simulink model "s_heli3d"  (R2022b)
settings: Solver=FixedStepAuto  StartTime=0.0  StopTime=50  FixedStep=0.05  RelTol=1e-3  EnableMultiTasking=on
values from neighbouring files (symbols this model uses):
  CMD_RATE_LIMIT = 45.0 * pi / 180    (= 0.785398163397)    [setup_lab_heli_3d.m]
  K = zeros(2,6)    [setup_lab_heli_3d.m]
  K_AMP = 3    [setup_lab_heli_3d.m]
  SAT_INT_ERR_ELEV = 7.5    [setup_lab_heli_3d.m]
  SAT_INT_ERR_TRAVEL = 7.5    [setup_lab_heli_3d.m]
  VMAX_AMP = 24    [setup_lab_heli_3d.m]
  VMAX_DAC = 10    [setup_lab_heli_3d.m]
undefined symbols (not defined in the file or in its folder): A, B, F, G, H, L_input, L_states, N, u_max_hat, u_min_hat, x_max_hat, x_min_hat
libraries: simulink_extras x6
settings Model: ExtModeTrigDuration=5000  Creator=MLevis  LastModifiedBy=START
settings SolverCC: AlgebraicLoopSolver=TrustRegion  PositivePriorityOrder=on
settings DataIOCC: LimitDataPoints=on  SaveFormat=Array  SignalLoggingSaveFormat=ModelDataLogs  ReturnWorkspaceOutputs=off
settings OptimizationCC: BooleanDataType=off  OptimizeBlockIOStorage=off  BufferReuse=off  ExpressionFolding=off  ExpressionDepthLimit=2147483647  LocalBlockOutputs=off  InitFltsAndDblsToZero=on
settings DebuggingCC: SaveWithParameterizedLinksMsg=none  UnderspecifiedInitializationDetection=Classic  MergeDetectMultiDrivingBlocksExec=none  SignalResolutionControl=TryResolveAllWithWarning  SolverPrmCheckMsg=warning  MultiTaskDSMMsg=warning  MultiTaskCondExecSysMsg=none  FcnCallInpInsideContextMsg=warning  UnconnectedInputMsg=warning  UnconnectedOutputMsg=warning  UnconnectedLineMsg=warning  StateNameClashWarn=warning  SFUnexpectedBacktrackingDiag=warning  SFNoUnconditionalDefaultTransitionDiag=warning  SFExecutionAtInitializationDiag=none  SFMachineParentedDataDiag=warning  ArithmeticOperatorsInVariantConditions=warning
settings HardwareCC: ProdBitPerPointer=32  ProdBitPerSizeT=32  ProdBitPerPtrDiffT=32  ProdWordSize=32  ProdHWDeviceType=Intel->x86-32 (Windows32)
settings ModelReferenceCC: EnableRefExpFcnMdlSchedulingChecks=on  PropagateSignalLabelsOutOfModel=off
settings RTWCC: Description=QUARC Win32 Target Using Toolchain  SystemTargetFile=quarc_windows.tlc  TemplateMakefile=quarc_default_tmf  Toolchain=QUARC windows | nmake (64-bit Windows)  BuildConfiguration=Faster Runs  DLArmComputeVersion=19.05
settings CodeAppCC: StateflowObjectComments=on
settings STFCustomTargetCC: ConcurrentExecutionCompliant=on  GRTInterface=on  UseToolchainInfoCompliant=on  SystemTargetFile=quarc_windows.tlc
settings GRTTargetCC: TargetLangStandard=C89/C90 (ANSI)  ParMdlRefBuildCompliant=off  CompOptLevelCompliant=off  CombineOutputUpdateFcns=off  MatFileLogging=off  CPPClassGenCompliant=off  GRTInterface=on  ExtMode=on  ExtModeMexFile=quarc_comm
settings ConfigComp: CovMetricSettings=dw  CovSaveCumulativeToWorkspaceVar=on  CovSaveSingleToWorkspaceVar=on

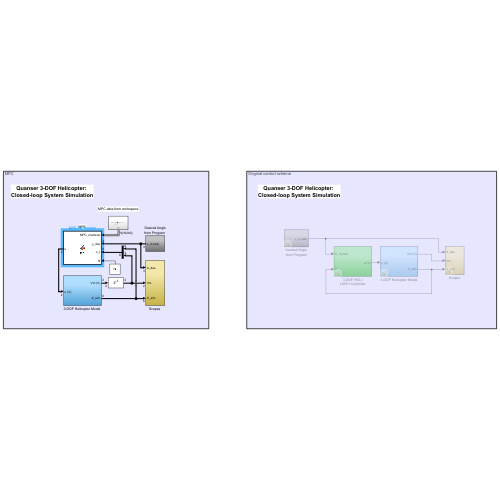
[thumbnail: Simulink's stored preview of the top-level diagram]
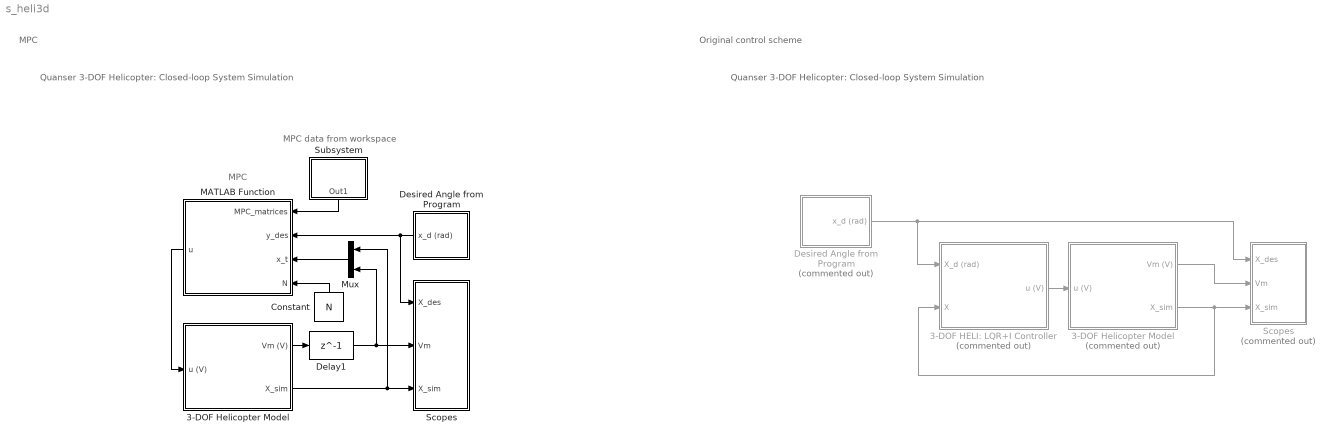
== system s_heli3d ==
  note: Original control scheme
  note: MPC
  note: MPC data from workspace
  note: MPC
  note: Quanser 3-DOF Helicopter:
      | Closed-loop System Simulation
  note: Quanser 3-DOF Helicopter:
      | Closed-loop System Simulation
  3-DOF HELI: LQR+I Controller : Subsystem  Commented=on  AncestorBlock=heli_2d_lib/2DOF HELI: FF+LQR+I Controller
      settings: LibrarySourceBlock=|
      | heli_2d_lib/2DOF HELI:
      | FF+LQR+I Controller
  3-DOF Helicopter Model : Subsystem  Commented=on
  "3-DOF Helicopter Model " : Subsystem
  Constant : Constant  Value=N
  Delay1 : Delay  DelayLength=1  InitialCondition=0
  Desired Angle from Program : Subsystem  Commented=on
  "Desired Angle from Program " : Subsystem
  MATLAB Function : MATLAB Function  Tag=MPC  Description=MPC  TreatAsAtomicUnit=on
  Mux : Mux  Inputs=2
  Scopes : Subsystem  Commented=on
  "Scopes " : Subsystem
  Subsystem : Subsystem
  wires:
  Desired Angle from Program/1(x_d (rad)) -> Scopes/1(X_des), 3-DOF HELI: LQR+I Controller/1(X_d (rad))
  3-DOF HELI: LQR+I Controller/1(u (V)) -> 3-DOF Helicopter Model/1(u (V))
  3-DOF Helicopter Model/2(X_sim) -> Scopes/3(X_sim), 3-DOF HELI: LQR+I Controller/2(X)
  3-DOF Helicopter Model/1(Vm (V)) -> Scopes/2(Vm)
  Mux/1 -> MATLAB Function/3(x_t)
  MATLAB Function/1(u) -> "3-DOF Helicopter Model "/1(u (V))
  "3-DOF Helicopter Model "/2(X_sim) -> Mux/1, "Scopes "/3(X_sim)
  "3-DOF Helicopter Model "/1(Vm (V)) -> Delay1/1
  "Desired Angle from Program "/1(x_d (rad)) -> MATLAB Function/2(y_des), "Scopes "/1(X_des)
  Subsystem/1(Out1) -> MATLAB Function/1(MPC_matrices)
  Constant/1 -> MATLAB Function/4(N)
  Delay1/1 -> Mux/2, "Scopes "/2(Vm)

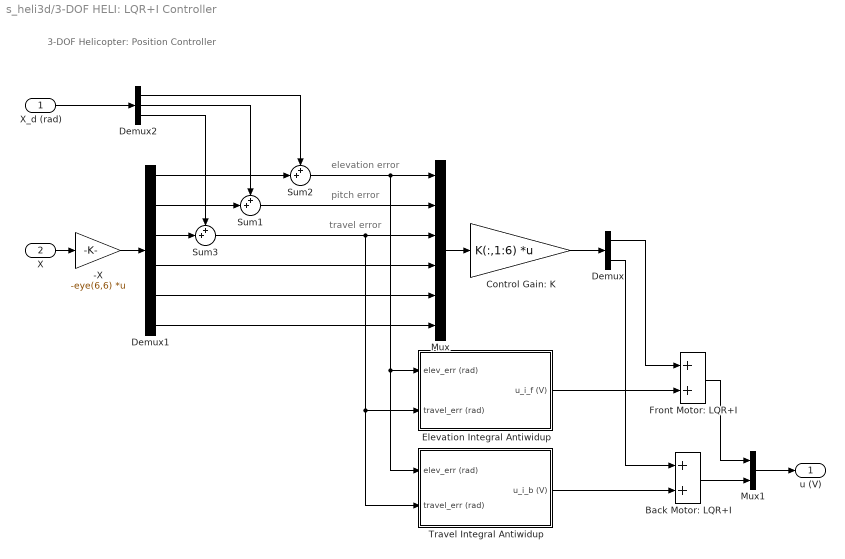
== system s_heli3d/3-DOF HELI: LQR+I Controller ==
  note: elevation error
  note: pitch error
  note: 3-DOF Helicopter: Position Controller
  note: travel error
  X_d (rad) : Inport
  X : Inport  Port=2
  -X : Gain  Gain=-eye(6,6)  Multiplication=Matrix(K*u)
  Back Motor: LQR+I : Sum
  Control Gain: K : Gain  Gain=K(:,1:6)  Multiplication=Matrix(K*u)
  Demux : Demux  Outputs=2
  Demux1 : Demux  Outputs=6
  Demux2 : Demux  Outputs=3
  Elevation Integral Antiwidup : Subsystem
  Front Motor: LQR+I : Sum
  Mux : Mux  Inputs=6
  Mux1 : Mux  Inputs=2
  Sum1 : Sum  Inputs=++|
  Sum2 : Sum  Inputs=++|
  Sum3 : Sum  Inputs=++|
  Travel Integral Antiwidup : Subsystem
  u (V) : Outport
  wires:
  Back Motor: LQR+I/1 -> Mux1/2
  Demux/1 -> Front Motor: LQR+I/1
  Demux/2 -> Back Motor: LQR+I/1
  Travel Integral Antiwidup/1(u_i_b (V)) -> Back Motor: LQR+I/2
  Elevation Integral Antiwidup/1(u_i_f (V)) -> Front Motor: LQR+I/2
  Demux1/2 -> Sum1/2
  Demux2/2 -> Sum1/1
  Demux2/1 -> Sum2/1
  X_d (rad)/1 -> Demux2/1
  Sum2/1 -> Mux/1, Elevation Integral Antiwidup/1(elev_err (rad)), Travel Integral Antiwidup/1(elev_err (rad))
  Demux1/1 -> Sum2/2
  X/1 -> -X/1
  Sum1/1 -> Mux/2
  -X/1 -> Demux1/1
  Mux/1 -> Control Gain: K/1
  Demux1/4 -> Mux/4
  Demux2/3 -> Sum3/1
  Demux1/3 -> Sum3/2
  Sum3/1 -> Mux/3, Elevation Integral Antiwidup/2(travel_err (rad)), Travel Integral Antiwidup/2(travel_err (rad))
  Demux1/5 -> Mux/5
  Demux1/6 -> Mux/6
  Control Gain: K/1 -> Demux/1
  Mux1/1 -> u (V)/1
  Front Motor: LQR+I/1 -> Mux1/1

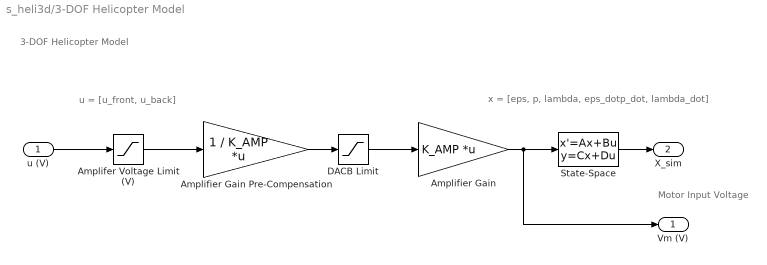
== system s_heli3d/3-DOF Helicopter Model ==
  note: x = [eps, p, lambda, eps_dotp_dot, lambda_dot]
  note: u = [u_front, u_back]
  note: Motor Input Voltage
  note: 3-DOF Helicopter Model
  u (V) : Inport
  Amplifer Voltage Limit (V) : Saturate  UpperLimit=VMAX_AMP  LowerLimit=-VMAX_AMP
  Amplifier Gain : Gain  Gain=K_AMP  Multiplication=Matrix(K*u)  SaturateOnIntegerOverflow=on  OutDataTypeStr=Inherit: Same as input  ParamDataTypeStr=Inherit: Same as input
  Amplifier Gain Pre-Compensation : Gain  Gain=1 / K_AMP  Multiplication=Matrix(K*u)  SaturateOnIntegerOverflow=on  OutDataTypeStr=Inherit: Same as input  ParamDataTypeStr=Inherit: Same as input
  DACB Limit : Saturate  UpperLimit=VMAX_DAC  LowerLimit=-VMAX_DAC
  State-Space : StateSpace  A=A  B=B  C=eye(6,6)  D=zeros(6,2)  InitialCondition=0
  Vm (V) : Outport
  X_sim : Outport  Port=2
  wires:
  u (V)/1 -> Amplifer Voltage Limit (V)/1
  Amplifier Gain/1 -> Vm (V)/1, State-Space/1
  State-Space/1 -> X_sim/1
  Amplifer Voltage Limit (V)/1 -> Amplifier Gain Pre-Compensation/1
  Amplifier Gain Pre-Compensation/1 -> DACB Limit/1
  DACB Limit/1 -> Amplifier Gain/1

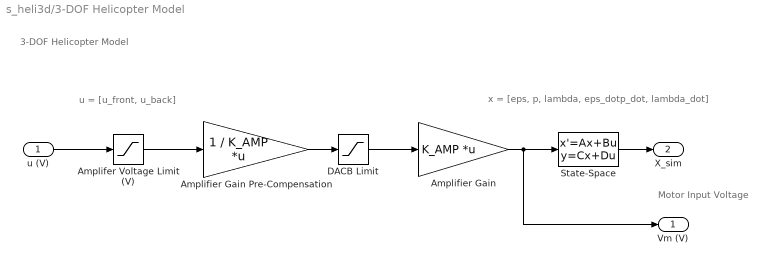
== system s_heli3d/3-DOF Helicopter Model  ==
  note: x = [eps, p, lambda, eps_dotp_dot, lambda_dot]
  note: u = [u_front, u_back]
  note: Motor Input Voltage
  note: 3-DOF Helicopter Model
  u (V) : Inport
  Amplifer Voltage Limit (V) : Saturate  UpperLimit=VMAX_AMP  LowerLimit=-VMAX_AMP
  Amplifier Gain : Gain  Gain=K_AMP  Multiplication=Matrix(K*u)  SaturateOnIntegerOverflow=on  OutDataTypeStr=Inherit: Same as input  ParamDataTypeStr=Inherit: Same as input
  Amplifier Gain Pre-Compensation : Gain  Gain=1 / K_AMP  Multiplication=Matrix(K*u)  SaturateOnIntegerOverflow=on  OutDataTypeStr=Inherit: Same as input  ParamDataTypeStr=Inherit: Same as input
  DACB Limit : Saturate  UpperLimit=VMAX_DAC  LowerLimit=-VMAX_DAC
  State-Space : StateSpace  A=A  B=B  C=eye(6,6)  D=zeros(6,2)  InitialCondition=0
  Vm (V) : Outport
  X_sim : Outport  Port=2
  wires:
  u (V)/1 -> Amplifer Voltage Limit (V)/1
  Amplifier Gain/1 -> Vm (V)/1, State-Space/1
  State-Space/1 -> X_sim/1
  Amplifer Voltage Limit (V)/1 -> Amplifier Gain Pre-Compensation/1
  Amplifier Gain Pre-Compensation/1 -> DACB Limit/1
  DACB Limit/1 -> Amplifier Gain/1

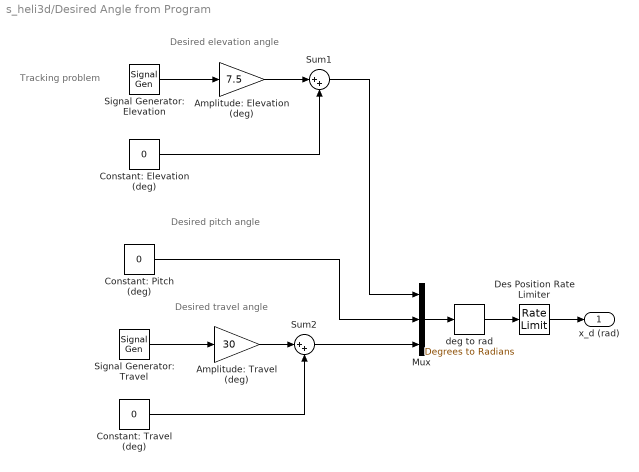
== system s_heli3d/Desired Angle from Program ==
  note: Tracking problem
  note: Desired elevation angle
  note: Desired travel angle
  note: Desired pitch angle
  Amplitude: Elevation (deg) : Gain  Gain=7.5
  Amplitude: Travel (deg) : Gain  Gain=30
  Constant: Elevation (deg) : Constant  Value=0
  Constant: Pitch (deg) : Constant  Value=0
  Constant: Travel (deg) : Constant  Value=0
  Des Position Rate Limiter : RateLimiter  RisingSlewLimit=CMD_RATE_LIMIT  FallingSlewLimit=-CMD_RATE_LIMIT  SampleTimeMode=inherited
  Mux : Mux  Inputs=3
  Signal Generator: Elevation : SignalGenerator  WaveForm=square  Frequency=0.04
  Signal Generator: Travel : SignalGenerator  WaveForm=square  Frequency=0.03
  Sum1 : Sum  Inputs=|++
  Sum2 : Sum  Inputs=|++
  deg to rad : simulink_extras/Transformations/Degrees to Radians
  x_d (rad) : Outport
  wires:
  Mux/1 -> deg to rad/1
  Constant: Elevation (deg)/1 -> Sum1/2
  Amplitude: Elevation (deg)/1 -> Sum1/1
  Signal Generator: Elevation/1 -> Amplitude: Elevation (deg)/1
  Constant: Travel (deg)/1 -> Sum2/2
  Amplitude: Travel (deg)/1 -> Sum2/1
  Signal Generator: Travel/1 -> Amplitude: Travel (deg)/1
  Sum2/1 -> Mux/3
  deg to rad/1 -> Des Position Rate Limiter/1
  Constant: Pitch (deg)/1 -> Mux/2
  Sum1/1 -> Mux/1
  Des Position Rate Limiter/1 -> x_d (rad)/1

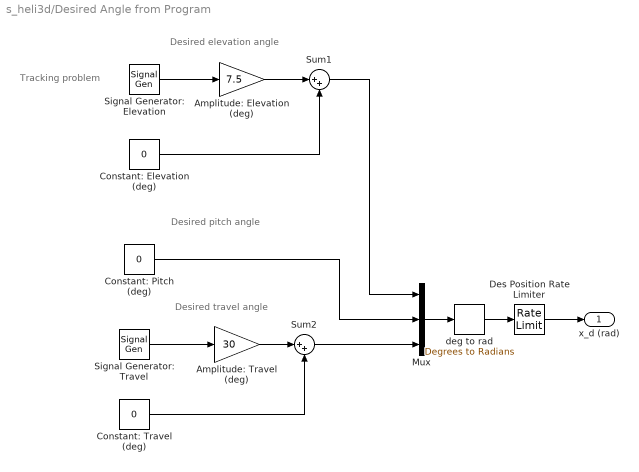
== system s_heli3d/Desired Angle from Program  ==
  note: Tracking problem
  note: Desired elevation angle
  note: Desired travel angle
  note: Desired pitch angle
  Amplitude: Elevation (deg) : Gain  Gain=7.5
  Amplitude: Travel (deg) : Gain  Gain=30
  Constant: Elevation (deg) : Constant  Value=0
  Constant: Pitch (deg) : Constant  Value=0
  Constant: Travel (deg) : Constant  Value=0
  Des Position Rate Limiter : RateLimiter  RisingSlewLimit=CMD_RATE_LIMIT  FallingSlewLimit=-CMD_RATE_LIMIT  SampleTimeMode=inherited
  Mux : Mux  Inputs=3
  Signal Generator: Elevation : SignalGenerator  WaveForm=square  Frequency=0.04
  Signal Generator: Travel : SignalGenerator  WaveForm=square  Frequency=0.03
  Sum1 : Sum  Inputs=|++
  Sum2 : Sum  Inputs=|++
  deg to rad : simulink_extras/Transformations/Degrees to Radians
  x_d (rad) : Outport
  wires:
  Mux/1 -> deg to rad/1
  Signal Generator: Elevation/1 -> Amplitude: Elevation (deg)/1
  Constant: Travel (deg)/1 -> Sum2/2
  Signal Generator: Travel/1 -> Amplitude: Travel (deg)/1
  Sum2/1 -> Mux/3
  Constant: Pitch (deg)/1 -> Mux/2
  Sum1/1 -> Mux/1
  Constant: Elevation (deg)/1 -> Sum1/2
  Amplitude: Elevation (deg)/1 -> Sum1/1
  deg to rad/1 -> Des Position Rate Limiter/1
  Des Position Rate Limiter/1 -> x_d (rad)/1
  Amplitude: Travel (deg)/1 -> Sum2/1

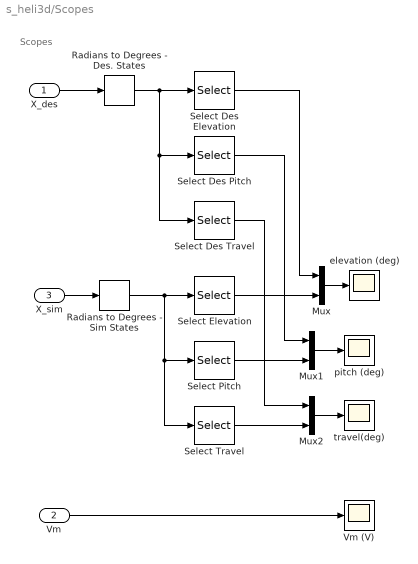
== system s_heli3d/Scopes ==
  note: Scopes
  X_des : Inport
  Vm : Inport  Port=2
  X_sim : Inport  Port=3
  Mux : Mux  Inputs=2
  Mux1 : Mux  Inputs=2
  Mux2 : Mux  Inputs=2
  Radians to Degrees - Des. States : simulink_extras/Transformations/Radians to Degrees
  Radians to Degrees - Sim States : simulink_extras/Transformations/Radians to Degrees
  Select Des Elevation : Selector  InputPortWidth=3  IndexOptions=Index vector (dialog)  Indices=1  OutputSizes=1
  Select Des Pitch : Selector  InputPortWidth=3  IndexOptions=Index vector (dialog)  Indices=2  OutputSizes=1
  Select Des Travel : Selector  InputPortWidth=3  IndexOptions=Index vector (dialog)  Indices=3  OutputSizes=1
  Select Elevation : Selector  InputPortWidth=6  IndexOptions=Index vector (dialog)  Indices=1  OutputSizes=1
  Select Pitch : Selector  InputPortWidth=6  IndexOptions=Index vector (dialog)  Indices=2  OutputSizes=1
  Select Travel : Selector  InputPortWidth=6  IndexOptions=Index vector (dialog)  Indices=3  OutputSizes=1
  Vm (V) : Scope
  elevation (deg) : Scope
  pitch (deg) : Scope
  travel(deg) : Scope
  wires:
  X_des/1 -> Radians to Degrees - Des. States/1
  X_sim/1 -> Radians to Degrees - Sim States/1
  Mux/1 -> elevation (deg)/1
  Mux1/1 -> pitch (deg)/1
  Vm/1 -> Vm (V)/1
  Radians to Degrees - Sim States/1 -> Select Elevation/1, Select Pitch/1, Select Travel/1
  Mux2/1 -> travel(deg)/1
  Select Elevation/1 -> Mux/2
  Select Pitch/1 -> Mux1/2
  Select Travel/1 -> Mux2/2
  Radians to Degrees - Des. States/1 -> Select Des Elevation/1, Select Des Pitch/1, Select Des Travel/1
  Select Des Elevation/1 -> Mux/1
  Select Des Pitch/1 -> Mux1/1
  Select Des Travel/1 -> Mux2/1

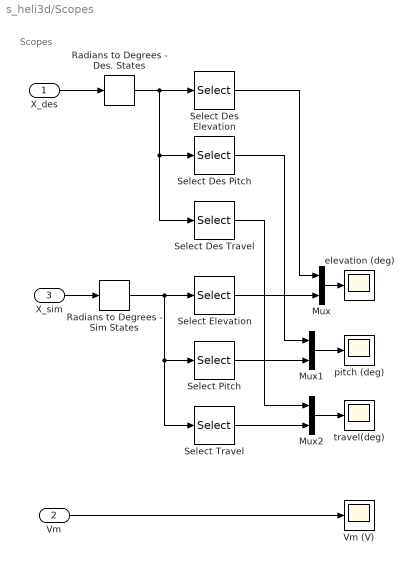
== system s_heli3d/Scopes  ==
  note: Scopes
  X_des : Inport
  Vm : Inport  Port=2
  X_sim : Inport  Port=3
  Mux : Mux  Inputs=2
  Mux1 : Mux  Inputs=2
  Mux2 : Mux  Inputs=2
  Radians to Degrees - Des. States : simulink_extras/Transformations/Radians to Degrees
  Radians to Degrees - Sim States : simulink_extras/Transformations/Radians to Degrees
  Select Des Elevation : Selector  InputPortWidth=3  IndexOptions=Index vector (dialog)  Indices=1  OutputSizes=1
  Select Des Pitch : Selector  InputPortWidth=3  IndexOptions=Index vector (dialog)  Indices=2  OutputSizes=1
  Select Des Travel : Selector  InputPortWidth=3  IndexOptions=Index vector (dialog)  Indices=3  OutputSizes=1
  Select Elevation : Selector  InputPortWidth=6  IndexOptions=Index vector (dialog)  Indices=1  OutputSizes=1
  Select Pitch : Selector  InputPortWidth=6  IndexOptions=Index vector (dialog)  Indices=2  OutputSizes=1
  Select Travel : Selector  InputPortWidth=6  IndexOptions=Index vector (dialog)  Indices=3  OutputSizes=1
  Vm (V) : Scope
  elevation (deg) : Scope
  pitch (deg) : Scope
  travel(deg) : Scope
  wires:
  X_des/1 -> Radians to Degrees - Des. States/1
  X_sim/1 -> Radians to Degrees - Sim States/1
  Mux/1 -> elevation (deg)/1
  Mux1/1 -> pitch (deg)/1
  Vm/1 -> Vm (V)/1
  Radians to Degrees - Sim States/1 -> Select Elevation/1, Select Pitch/1, Select Travel/1
  Mux2/1 -> travel(deg)/1
  Select Elevation/1 -> Mux/2
  Select Pitch/1 -> Mux1/2
  Select Travel/1 -> Mux2/2
  Radians to Degrees - Des. States/1 -> Select Des Elevation/1, Select Des Pitch/1, Select Des Travel/1
  Select Des Elevation/1 -> Mux/1
  Select Des Pitch/1 -> Mux1/1
  Select Des Travel/1 -> Mux2/1

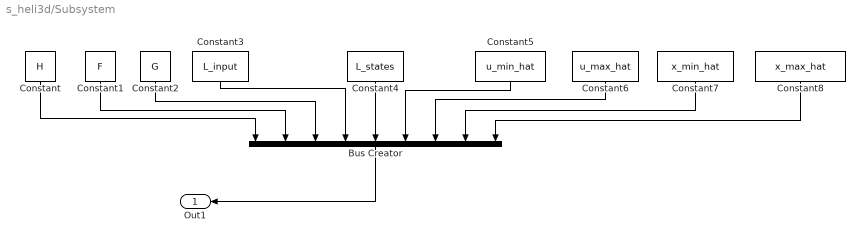
== system s_heli3d/Subsystem ==
  Bus Creator : BusCreator  Inputs=9  OutDataTypeStr=Bus: myBus
      settings: InheritFromInputs=off
  Constant : Constant  Value=H
  Constant1 : Constant  Value=F
  Constant2 : Constant  Value=G
  Constant3 : Constant  Value=L_input
  Constant4 : Constant  Value=L_states
  Constant5 : Constant  Value=u_min_hat
  Constant6 : Constant  Value=u_max_hat
  Constant7 : Constant  Value=x_min_hat
  Constant8 : Constant  Value=x_max_hat
  Out1 : Outport
  wires:
  Constant/1 -> Bus Creator/1
  Constant5/1 -> Bus Creator/6
  Constant3/1 -> Bus Creator/4
  Constant4/1 -> Bus Creator/5
  Constant2/1 -> Bus Creator/3
  Constant6/1 -> Bus Creator/7
  Bus Creator/1 -> Out1/1
  Constant1/1 -> Bus Creator/2
  Constant7/1 -> Bus Creator/8
  Constant8/1 -> Bus Creator/9

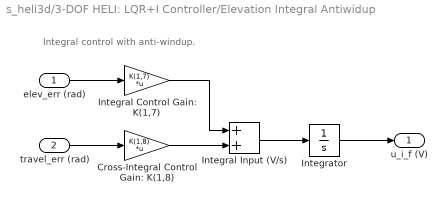
== system s_heli3d/3-DOF HELI: LQR+I Controller/Elevation Integral Antiwidup ==
  note: Integral control with anti-windup.
  elev_err (rad) : Inport
  travel_err (rad) : Inport  Port=2
  Cross-Integral Control Gain: K(1,8) : Gain  Gain=K(1,8)  Multiplication=Matrix(K*u)
  Integral Control Gain: K(1,7) : Gain  Gain=K(1,7)  Multiplication=Matrix(K*u)
  Integral Input (V/s) : Sum
  Integrator : Integrator  LimitOutput=on  UpperSaturationLimit=SAT_INT_ERR_ELEV  LowerSaturationLimit=-SAT_INT_ERR_ELEV
  u_i_f (V) : Outport
  wires:
  Cross-Integral Control Gain: K(1,8)/1 -> Integral Input (V/s)/2
  Integral Control Gain: K(1,7)/1 -> Integral Input (V/s)/1
  travel_err (rad)/1 -> Cross-Integral Control Gain: K(1,8)/1
  elev_err (rad)/1 -> Integral Control Gain: K(1,7)/1
  Integral Input (V/s)/1 -> Integrator/1
  Integrator/1 -> u_i_f (V)/1

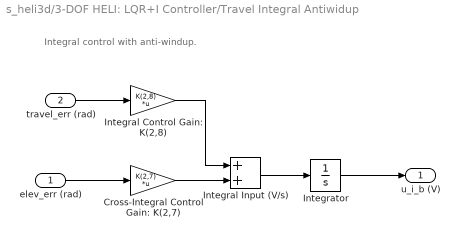
== system s_heli3d/3-DOF HELI: LQR+I Controller/Travel Integral Antiwidup ==
  note: Integral control with anti-windup.
  elev_err (rad) : Inport
  travel_err (rad) : Inport  Port=2
  Cross-Integral Control Gain: K(2,7) : Gain  Gain=K(2,7)  Multiplication=Matrix(K*u)
  Integral Control Gain: K(2,8) : Gain  Gain=K(2,8)  Multiplication=Matrix(K*u)
  Integral Input (V/s) : Sum
  Integrator : Integrator  LimitOutput=on  UpperSaturationLimit=SAT_INT_ERR_TRAVEL  LowerSaturationLimit=-SAT_INT_ERR_TRAVEL
  u_i_b (V) : Outport
  wires:
  Cross-Integral Control Gain: K(2,7)/1 -> Integral Input (V/s)/2
  Integral Control Gain: K(2,8)/1 -> Integral Input (V/s)/1
  travel_err (rad)/1 -> Integral Control Gain: K(2,8)/1
  elev_err (rad)/1 -> Cross-Integral Control Gain: K(2,7)/1
  Integral Input (V/s)/1 -> Integrator/1
  Integrator/1 -> u_i_b (V)/1

== matlab function s_heli3d/MATLAB Function ==
  data: MPC_matrices input; y_des input; x_t input; u output; N input
function u = fcn(MPC_matrices, y_des, x_t, N)

H = MPC_matrices.H;
F = MPC_matrices.F;
G = MPC_matrices.G;
L_input = MPC_matrices.L_input;
L_states = MPC_matrices.L_states;
u_min_hat = MPC_matrices.u_min_hat;
u_max_hat = MPC_matrices.u_max_hat;
x_min_hat = MPC_matrices.x_min_hat;
x_max_hat = MPC_matrices.x_max_hat;
y_des_hat = repmat(y_des, N,1);

P = [u_max_hat - L_input * x_t;
     x_max_hat - L_states * x_t;
     L_input*x_t - u_min_hat;
     L_states*x_t - x_min_hat];

f = ([x_t.' y_des_hat.']*F).';

H = 0.5*(H+H');

x0 = zeros(N*2, 1);                      % Initial guess
opts = optimoptions('quadprog', 'Algorithm', 'active-set');
delta_u_opt = quadprog(H, f, G, P, [], [], [], [], x0, opts);

u = x_t(7:8)+delta_u_opt(1:2);
